simulink model "SysModelling_Lab2"  (R2023a)
settings: Solver=VariableStepAuto  StartTime=0.0  StopTime=10.0  FixedStep=0.001  MaxStep=0.2  RelTol=1e-3
libraries: simulink x1
settings Model: Creator=pks11  LastModifiedBy=pks11

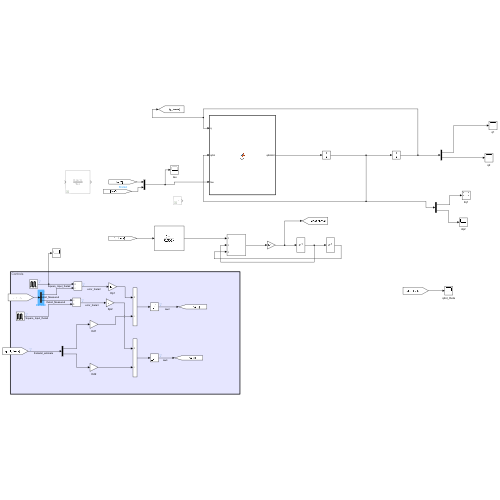
[thumbnail: Simulink's stored preview of the top-level diagram]
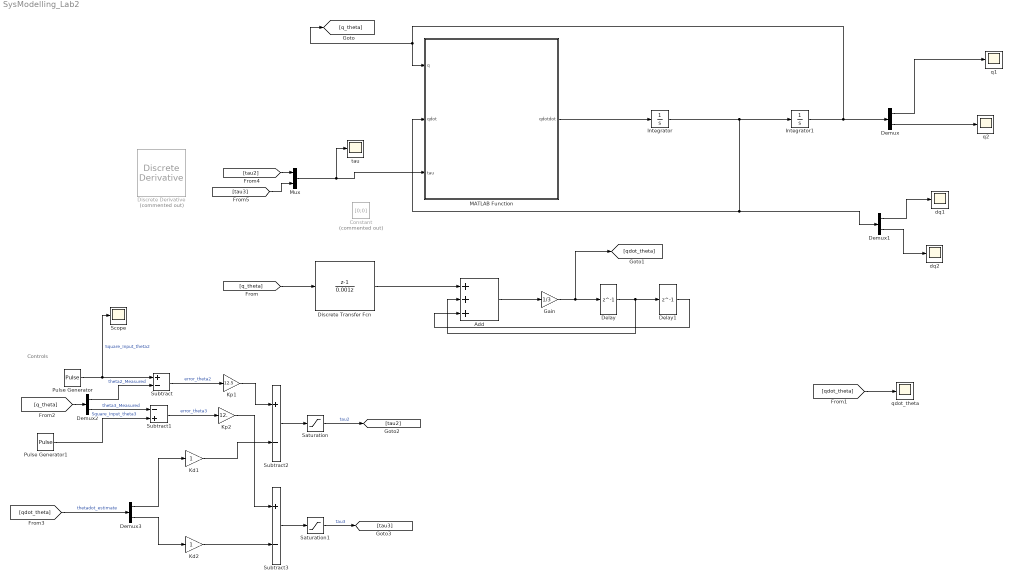
== system SysModelling_Lab2 ==
  note: Controls
  Add : Sum  Inputs=+++
  Constant : Constant  Commented=on  Value=[0;0]
  Delay : Delay  DelayLength=1  SampleTime=0.001
  Delay1 : Delay  DelayLength=1  SampleTime=0.001
  Demux{,1..3} (4 alike) : Demux  Outputs=2
  Discrete Transfer Fcn : DiscreteTransferFcn  Numerator=[1,-1]  Denominator=[0.001,0]  SampleTime=0.001
  Discrete Derivative : simulink/Discrete/Discrete Derivative  Commented=on  gainval=1.0  ICPrevScaledInput=0.001  OutMin=[]  OutMax=[]  OutDataType=fixdt(1, 16)  OutScaling=2^-10  DoSatur=off
  Gain : Gain  Gain=1/3
  Integrator : Integrator  InitialCondition=[0;0]
  Integrator1 : Integrator  InitialCondition=[pi;pi/2]
  Kd1 : Gain
  Kd2 : Gain
  Kp1 : Gain  Gain=12.5
  Kp2 : Gain  Gain=12.
  MATLAB Function : MATLAB Function  TreatAsAtomicUnit=on
  Mux : Mux  Inputs=2
  Pulse Generator : DiscretePulseGenerator  PulseType=Time based  Amplitude=pi/6  PulseWidth=50
  Pulse Generator1 : DiscretePulseGenerator  PulseType=Time based  Amplitude=pi/6  PulseWidth=50
  Saturation : Saturate  UpperLimit=5  LowerLimit=-5
  Saturation1 : Saturate  UpperLimit=5  LowerLimit=-5
  Scope : Scope
  Subtract : Sum  Inputs=+-
  Subtract1 : Sum  Inputs=-+
  Subtract2 : Sum  Inputs=+-
  Subtract3 : Sum  Inputs=+-
  dq1 : Scope
  dq2 : Scope
  q1 : Scope
  q2 : Scope
  qdot_theta : Scope
  tau : Scope
  wires:
  MATLAB Function/1(qdotdot) -> Integrator/1
  Integrator1/1 -> [q_theta], MATLAB Function/1(q), Demux/1
  Mux/1 -> tau/1, MATLAB Function/3(tau)
  Integrator/1 -> MATLAB Function/2(qdot), Demux1/1, Integrator1/1
  Demux/1 -> q1/1
  Demux/2 -> q2/1
  Demux1/1 -> dq1/1
  Demux1/2 -> dq2/1
  [q_theta] -> Discrete Transfer Fcn/1
  Add/1 -> Gain/1
  Gain/1 -> [qdot_theta], Delay/1
  Discrete Transfer Fcn/1 -> Add/1
  Delay/1 -> Add/2, Delay1/1
  Delay1/1 -> Add/3
  [qdot_theta] -> qdot_theta/1
  Pulse Generator1/1 -> Subtract1/2  "Square_Input_theta3"
  Pulse Generator/1 -> Scope/1, Subtract/1  "Square_Input_theta2"
  [q_theta] -> Demux2/1
  Demux2/1 -> Subtract/2  "theta2_Measured"
  Demux2/2 -> Subtract1/1  "theta3_Measured"
  Subtract/1 -> Kp1/1  "error_theta2"
  Subtract1/1 -> Kp2/1  "error_theta3"
  [qdot_theta] -> Demux3/1  "thetadot_estimate"
  Demux3/1 -> Kd1/1
  Demux3/2 -> Kd2/1
  Kp1/1 -> Subtract2/1
  Kd1/1 -> Subtract2/2
  Kp2/1 -> Subtract3/1
  Kd2/1 -> Subtract3/2
  Subtract2/1 -> Saturation/1
  [tau2] -> Mux/1
  [tau3] -> Mux/2
  Saturation/1 -> [tau2]  "tau2"
  Subtract3/1 -> Saturation1/1
  Saturation1/1 -> [tau3]  "tau3"

== matlab function SysModelling_Lab2/MATLAB Function ==
  data: q input; qdotdot output; qdot input; tau input
function qdotdot = fcn(q,qdot,tau)
%parameters (PWM units*s2/m)
p1 = 0.0300;
p2 = 0.0128;
p3 = 0.0076;
p4 = 0.0753;
p5 = 0.0298;
g = 9.81;
qdotdot = [0;0];

D_theta = [p1, -p3*sin(q(2) - q(1));
            -p3*sin(q(2) - q(1))  p2 ];

C_thetathetadot = [0,  -p3*cos(q(2) - q(1))*qdot(2);
                    p3*cos(q(2) - q(1))*qdot(1),  0 ];

G_theta = [-p4*g*sin(q(1));
            -p5*g*cos(q(2))];

D_thetainv = inv(D_theta);

qdotdot = D_thetainv*tau - D_thetainv*C_thetathetadot*qdot - D_thetainv*G_theta;

y = qdotdot;
